simulink model "Simulink_Lab2"  (R2014a)
settings: Solver=ode45  StartTime=0.0  StopTime=10.0  RelTol=1e-3
settings Model: Creator=Omar Emad  LastModifiedBy=Omar Emad

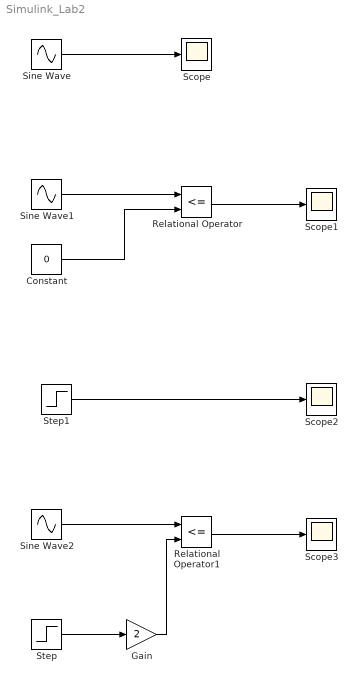
== system Simulink_Lab2 ==
  Constant : Constant  Value=0
  Gain : Gain  Gain=2
  Relational Operator : RelationalOperator  Operator=<=  OutDataTypeStr=boolean
  Relational Operator1 : RelationalOperator  Operator=<=  OutDataTypeStr=boolean
  Scope{,1..3} (4 alike) : Scope
      Scope2 settings: SaveName=ScopeData2
      Scope3 settings: SaveName=ScopeData3
  Sine Wave : Sin  SampleTime=0
  Sine Wave1 : Sin  SampleTime=0
  Sine Wave2 : Sin  SampleTime=0
  Step : Step  Time=2  SampleTime=0
  Step1 : Step  Time=2  SampleTime=0
  wires:
  Sine Wave/1 -> Scope/1
  Sine Wave1/1 -> Relational Operator/1
  Relational Operator/1 -> Scope1/1
  Constant/1 -> Relational Operator/2
  Step/1 -> Gain/1
  Sine Wave2/1 -> Relational Operator1/1
  Relational Operator1/1 -> Scope3/1
  Gain/1 -> Relational Operator1/2
  Step1/1 -> Scope2/1
